simulink model "Original_example1_cs"  (R2018b)
settings: Solver=ode5  StartTime=0.0  StopTime=inf  FixedStep=1/20  RelTol=1e-3
PreLoadFcn:
  | mbxruntime.callbacks.PreLoadFcn(bdroot);
PostLoadFcn:
  | mbxruntime.callbacks.PostLoadFcn(bdroot);
InitFcn:
  | mbxruntime.callbacks.InitFcn(bdroot);
StartFcn:
  | mbxruntime.callbacks.StartFcn(bdroot);
StopFcn:
  | mbxruntime.callbacks.StopFcn(bdroot);
model workspace: external: MAT-File example1_cs_hws.mat (data not in the file)
undefined symbols (not defined in the file or in its folder): Broadcast, CameraTimestamp, Confidence, ConfidenceType, DiscIntNeverNeededParam, ErrorCode, Header, Height, Id, Id_SL_Info, InitImageOutputDir, Length, LidarTimestamp, PerceptionObstacle, PerceptionObstacle_SL_Info, PolygonPoint, PolygonPoint_SL_Info, Pose, Position, RadarTimestamp, S, SequenceNum, Theta, Timestamp, TimestampSec, TrackingTime, Type, Velocity, warningInitialVelocity, Waypoint, Waypoint_SL_Info, Width, X, x0, Y, Z
libraries: simulink x27, PreScanSimulinkLibrary x14, robotlib x12, simulink_extras x5, robotcorelib x2
(part 1 of 5)
CloseFcn:
  | mbxruntime.callbacks.CloseFcn(bdroot);
settings Model: Creator=PRESCAN  LastModifiedBy=im-lab
settings DataIOCC: LimitDataPoints=on  SaveFormat=Array  SignalLoggingSaveFormat=ModelDataLogs
settings OptimizationCC: ExpressionDepthLimit=2147483647  InitFltsAndDblsToZero=on  LifeSpan=inf
settings DebuggingCC: SaveWithParameterizedLinksMsg=none  UnderspecifiedInitializationDetection=Classic  MergeDetectMultiDrivingBlocksExec=none  SignalResolutionControl=TryResolveAllWithWarning  MultiTaskDSMMsg=warning  MultiTaskCondExecSysMsg=none  FcnCallInpInsideContextMsg=warning  StateNameClashWarn=warning  SFUnexpectedBacktrackingDiag=warning  SFNoUnconditionalDefaultTransitionDiag=warning  SFExecutionAtInitializationDiag=none
settings HardwareCC: ProdBitPerPointer=32  ProdBitPerSizeT=32  ProdBitPerPtrDiffT=32  ProdLargestAtomicFloat=None  ProdIntDivRoundTo=Undefined  ProdEndianess=Unspecified  ProdWordSize=32  ProdHWDeviceType=32-bit Generic
settings ModelReferenceCC: UpdateModelReferenceTargets=IfOutOfDate  PropagateSignalLabelsOutOfModel=off
settings SFSimCC: SimUseLocalCustomCode=off  SimParseCustomCode=off
settings SFSimCC: SimCustomHeaderCode=|
  | #include "prescan.h"
  | #include "prescan_platform.h"
settings RTWCC: RTWUseLocalCustomCode=off
settings CodeAppCC: StateflowObjectComments=on
settings GRTTargetCC: TargetFcnLib=ansi_tfl_tmw.mat  TargetLangStandard=C89/C90 (ANSI)  GeneratePreprocessorConditionals=Disable all  CombineOutputUpdateFcns=off  GRTInterface=on
settings ConfigComp: CovMetricSettings=dw  CovHtmlReporting=on  CovSaveCumulativeToWorkspaceVar=on  CovSaveSingleToWorkspaceVar=on  CovExternalEMLEnable=off

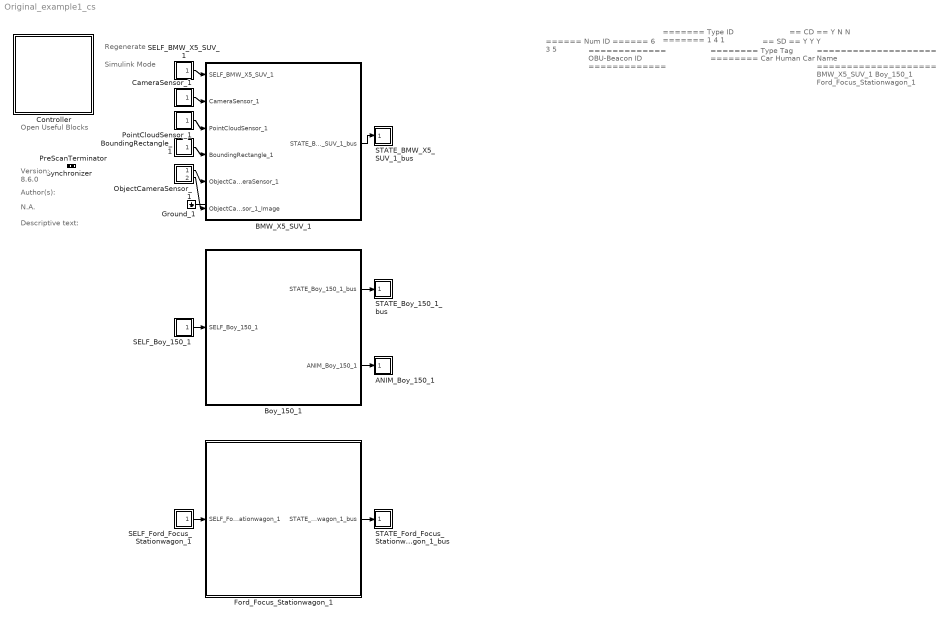
== system Original_example1_cs ==
  note: Regenerate
  note: Simulink Mode
  note: Open Useful Blocks
  note: 8.6.0
  note: Version:
  note: Author(s):
  note: N.A.
  note: Descriptive text:
  note: ======
      | Num ID
      | ======
      | 6
      | 3
      | 5
  note: =============
      | OBU-Beacon ID
      | =============
  note: =======
      | Type ID
      | =======
      | 1
      | 4
      | 1
  note: ========
      | Type Tag
      | ========
      | Car
      | Human
      | Car
  note: ==
      | SD
      | ==
      | Y
      | Y
      | Y
  note: ==
      | CD
      | ==
      | Y
      | N
      | N
  note: ====================
      | Name
      | ====================
      | BMW_X5_SUV_1
      | Boy_150_1
      | Ford_Focus_Stationwagon_1
  ANIM_Boy_150_1 : Subsystem  Tag=actuator/AnimationOutport  Priority=0  LoadFcn=load('PreScanAnimActuatorData.mat')  mask(PreScan Sink Block: State Animation){}
      mask help: The Human Animation port allows the human to walk, run or bend
      settings: OpenFcn=open_system([gcb '/Actuator'],'mask')
      mask Help: eval('openHelp(239)')
      mask Display: image(imread('HumanAnimated.jpg'))
  BMW_X5_SUV_1 : Subsystem  Tag=WorldObjectSubSystem  InitFcn=UniqueId = '35';
      mask init:
      | modelPath = GenericModelHelper.getGenericModelFilePath('ModelDepo','Vehicles\BMW_X5\BMW_X5.pgmb','cea918691563e9ae3e6a88ec95e6726a');imagePath = GenericModelHelper.getCompilationPicture(modelPath, 'BMW_X5_HighPoly.png');
      mask Display: image(imread(imagePath));color('white');text(0, 0, ' ID=6\n')
  BoundingRectangle_1 : Subsystem  Tag=sensor/BRS  Priority=3  LoadFcn=load('PrescanBRSData.mat');load('PrescanBRSMessage.mat')  mask(PreScan Source Block: Bounding Rectangle Sensor){}
      mask help: The Bounding Rectangle Sensor provides information of whereabouts of objects in images.
      settings: OpenFcn=open_system([gcb '/Sensor'],'mask')
      mask Help: eval('openHelp(1462)')
      mask Display: image(imread('BoundingRectangleSensorSL.png'))
  Boy_150_1 : Subsystem  Tag=WorldObjectSubSystem  InitFcn=UniqueId = '120';
      mask init:
      | modelPath = GenericModelHelper.getGenericModelFilePath('ModelDepo','Humans\Boy_150\Boy_150.pgmb','841f6aedbf99f0bd20b712839b1c33a7');imagePath = GenericModelHelper.getCompilationPicture(modelPath, 'Boy_150.png');
      mask Display: image(imread(imagePath));color('white');text(0, 0, ' ID=3\n')
  CameraSensor_1 : Subsystem  Tag=sensor/Camera/CameraSensor  Priority=3  mask(PreScan Source Block: Camera Sensor){}
      mask help: The Camera Sensor provides a color or monochrome image.
      settings: OpenFcn=open_system([gcb '/Sensor'],'mask')
      mask Help: eval('openHelp(457)')
      mask Display: image(imread('CameraSensor.png'))
  Controller : Subsystem  Description=193591AABAB723D448F28EC02D1309BC2290EA2C51FE96CBCBC842FCD2A763E3  Priority=-1  LoadFcn=load PreScanControllerData  mask(PreScan Simulation Controller){prescanversion='8.6.0', ModelReferencing=off, TimeStep=1/20, ControlMode=0, PreScanExecutionMode=on, ControllerCount=0, ControllerIndex=0, ControllerOptions=''}
      mask prompts: prescanversion "PreScan Version"; ModelReferencing "Use Model Referencing"; TimeStep "Upload Period [s]"; ControlMode "Control Mode"; PreScanExecutionMode "Execution Mode"; ControllerCount "Controller Count"; ControllerIndex "Controller Index"; ControllerOptions "Controller Options"
      mask help:
      | Please do not remove this block from the compilation sheet,
      | as it connects the model to the PreScan environment.
      mask init:
      | model = bdroot(gcb);
      | ExperimentFile = mbxruntime.findExperimentFile(model,true); %relative path
      | 
      | [d1, d2, d3, prescandata] = prescan_Settings();
      | ModelDepo = fullfile(prescandata,'ModelDepo'); 
      | 
      | RTmode = mbxruntime.getRTMode(model);
      | 
      | SimulationMode = get_param(bdroot,'SimulationMode');
      | if strcmp(SimulationMode, 'rapid-accelerator')
      |     SimulationMode = 'external';
      | end
      | TargetName = get_param(bdroot,'SystemTargetFile');
      settings: ModelCloseFcn=assignin('base',['model_closed_' bdroot],true);
      mask Help: eval('openHelp(812)')
      mask Display: image(imread('prescanlogo.ico'))
  Ford_Focus_Stationwagon_1 : Subsystem  Tag=WorldObjectSubSystem  InitFcn=UniqueId = '232';
      mask init:
      | modelPath = GenericModelHelper.getGenericModelFilePath('ModelDepo','Vehicles\Ford_Focus_Wagon\Ford_Focus_Wagon.pgmb','9f2f84850ce6f49365560c3439563633');imagePath = GenericModelHelper.getCompilationPicture(modelPath, 'Ford_Focus_Wagon_HighPoly.png');
      mask Display: image(imread(imagePath));color('white');text(0, 0, ' ID=5\n')
  Ground_1 : Ground
  ObjectCameraSensor_1 : Subsystem  Tag=sensor/ObjectCamera/data  Priority=3  LoadFcn=load('PrescanOCSData.mat');load('PrescanOCSMessage.mat')  mask(PreScan Source Block: Object Camera Sensor){}
      mask help: The Object Camera Sensor provides information on objects locations.
      settings: OpenFcn=open_system([gcb '/Sensor'],'mask')
      mask Help: eval('openHelp(2401)')
      mask Display: image(imread('ObjectCameraSensorSL.png'))
  PointCloudSensor_1 : Subsystem  Tag=sensor/PointCloudInport  Priority=3  mask(PreScan Source Block: Point Cloud Sensor){}
      mask help: The Point Cloud Sensor provides XYZ positions relative to the sensor
      settings: OpenFcn=open_system([gcb '/Sensor'],'mask')
      mask Help: eval('openHelp(6400)')
      mask Display: image(imread('PointCloudSensorSL.png'))
  PreScanTerminator : Subsystem  Tag=PreScanTerminator  Priority=999  LoadFcn=load PrescanTerminatorData  mask(PreScan Simulation Terminator){TimeStep=1/20}
      mask prompts: TimeStep "Upload Period [s]"
      mask help:
      | Please do not remove this block from the compilation sheet as it
      | connects the model to the PreScan environment.
      mask Help: eval('openHelp(812)')
      mask Display: image(imread('prescanlogo.ico'))
  SELF_BMW_X5_SUV_1 : Subsystem  Tag=sensor/SelfPort  Priority=3  LoadFcn=load('PreScanSelfSensorData.mat')  mask(PreScan Source Block: SELF){}
      mask help:
      | The SELF port shows (state) information of the actor itself. The outputs are position in the experiment's axis system and the GPS coordinates, and the object's absolute velocity and compass heading.
      |
      | For more information, please click Help.
      settings: OpenFcn=open_system([gcb '/Sensor'],'mask')
      mask Help: eval('openHelp(462)')
      mask Display: image(imread('GPS.png'))
  SELF_Boy_150_1 : Subsystem  Tag=sensor/SelfPort  Priority=3  LoadFcn=load('PreScanSelfSensorData.mat')  mask(PreScan Source Block: SELF){}
      mask help:
      | The SELF port shows (state) information of the actor itself. The outputs are position in the experiment's axis system and the GPS coordinates, and the object's absolute velocity and compass heading.
      |
      | For more information, please click Help.
      settings: OpenFcn=open_system([gcb '/Sensor'],'mask')
      mask Help: eval('openHelp(462)')
      mask Display: image(imread('GPS.png'))
  SELF_Ford_Focus_Stationwagon_1 : Subsystem  Tag=sensor/SelfPort  Priority=3  LoadFcn=load('PreScanSelfSensorData.mat')  mask(PreScan Source Block: SELF){}
      mask help:
      | The SELF port shows (state) information of the actor itself. The outputs are position in the experiment's axis system and the GPS coordinates, and the object's absolute velocity and compass heading.
      |
      | For more information, please click Help.
      settings: OpenFcn=open_system([gcb '/Sensor'],'mask')
      mask Help: eval('openHelp(462)')
      mask Display: image(imread('GPS.png'))
  STATE_BMW_X5_SUV_1_bus : Subsystem  Tag=actuator/StatePort  Priority=0  LoadFcn=load('PreScanStateActuatorData.mat')  mask(PreScan Sink Block: State){}
      mask help:
      | The Actor State contains a vector signal of size (9x1), containing the following signals:
      |
      | -  Position    	(x,y,z)             	[m]
      | -  Velocity    	(vx,vy,vz)         	[m/s]
      | -  Angles       	(Roll, Pitch, Yaw)	[rad]
      |
      | The Actor state is defined in the global axis system.
      | The state is superponed on the Initial position defined in the GUI.
      |
      | For more information, please click Help.
      settings: OpenFcn=open_system([gcb '/Actuator'],'mask')
      mask Help: eval('openHelp(222)')
      mask Display: image(imread('State.png'))
  STATE_Boy_150_1_bus : Subsystem  Tag=actuator/StatePort  Priority=0  LoadFcn=load('PreScanStateActuatorData.mat')  mask(PreScan Sink Block: State){}
      mask help:
      | The Actor State contains a vector signal of size (9x1), containing the following signals:
      |
      | -  Position    	(x,y,z)             	[m]
      | -  Velocity    	(vx,vy,vz)         	[m/s]
      | -  Angles       	(Roll, Pitch, Yaw)	[rad]
      |
      | The Actor state is defined in the global axis system.
      | The state is superponed on the Initial position defined in the GUI.
      |
      | For more information, please click Help.
      settings: OpenFcn=open_system([gcb '/Actuator'],'mask')
      mask Help: eval('openHelp(222)')
      mask Display: image(imread('State.png'))
  STATE_Ford_Focus_Stationwagon_1_bus : Subsystem  Tag=actuator/StatePort  Priority=0  LoadFcn=load('PreScanStateActuatorData.mat')  mask(PreScan Sink Block: State){}
      mask help:
      | The Actor State contains a vector signal of size (9x1), containing the following signals:
      |
      | -  Position    	(x,y,z)             	[m]
      | -  Velocity    	(vx,vy,vz)         	[m/s]
      | -  Angles       	(Roll, Pitch, Yaw)	[rad]
      |
      | The Actor state is defined in the global axis system.
      | The state is superponed on the Initial position defined in the GUI.
      |
      | For more information, please click Help.
      settings: OpenFcn=open_system([gcb '/Actuator'],'mask')
      mask Help: eval('openHelp(222)')
      mask Display: image(imread('State.png'))
  Synchronizer : Subsystem  Tag=PreScanSynchronizer  Priority=1  LoadFcn=load PrescanSynchronizeData  mask(PreScan Simulation Core Block){TimeStep=1/20}
      mask prompts: TimeStep "Timestep [s]"
      mask help:
      | Please do not remove this block from the PreScan compilation sheet,
      | as it contains essential configuration parameters for a PreScan simulation.
      settings: DeleteFcn=PreScanBlockDeleteFcn;
      mask Display: image(imread('prescanlogo.ico'))
  wires:
  BMW_X5_SUV_1/1(STATE_BMW_X5_SUV_1_bus) -> STATE_BMW_X5_SUV_1_bus/1(STATE_BMW_X5_SUV_1_bus)
  SELF_BMW_X5_SUV_1/1(SELF_BMW_X5_SUV_1) -> BMW_X5_SUV_1/1(SELF_BMW_X5_SUV_1)
  CameraSensor_1/1(CameraSensor_1) -> BMW_X5_SUV_1/2(CameraSensor_1)
  BoundingRectangle_1/1(BoundingRectangle_1) -> BMW_X5_SUV_1/4(BoundingRectangle_1)
  ObjectCameraSensor_1/1(ObjectCameraSensor_1) -> BMW_X5_SUV_1/5(ObjectCameraSensor_1)
  ObjectCameraSensor_1/2(ObjectCameraSensor_1_Image) -> BMW_X5_SUV_1/6(ObjectCameraSensor_1_Image)
  Boy_150_1/1(STATE_Boy_150_1_bus) -> STATE_Boy_150_1_bus/1(STATE_Boy_150_1_bus)
  Boy_150_1/2(ANIM_Boy_150_1) -> ANIM_Boy_150_1/1(ANIM_Boy_150_1)
  SELF_Boy_150_1/1(SELF_Boy_150_1) -> Boy_150_1/1(SELF_Boy_150_1)
  Ford_Focus_Stationwagon_1/1(STATE_Ford_Focus_Stationwagon_1_bus) -> STATE_Ford_Focus_Stationwagon_1_bus/1(STATE_Ford_Focus_Stationwagon_1_bus)
  SELF_Ford_Focus_Stationwagon_1/1(SELF_Ford_Focus_Stationwagon_1) -> Ford_Focus_Stationwagon_1/1(SELF_Ford_Focus_Stationwagon_1)
  PointCloudSensor_1/1(PointCloudSensor_1) -> BMW_X5_SUV_1/3(PointCloudSensor_1)
  Ground_1/1 -> ?

== system Original_example1_cs/ANIM_Boy_150_1 ==
  ANIM_Boy_150_1 : Inport  Tag=inport/AnimationOutport  OutDataTypeStr=Bus: PRESCAN_ANIMACTUATORDATA  PortDimensions=1  SampleTime=1/20  BusOutputAsStruct=on
  Actuator : S-Function  FunctionName=sfun_AnimActuator  Parameters=UniqueID, TimeStep  SFunctionDeploymentMode=off  EnableBusSupport=off  mask(PreScan Sink Block: State Animation){UniqueID=120, TimeStep=1/20}
      mask prompts: UniqueID "Auto-Assigned: Unique ID"; TimeStep "Auto-Assigned: Upload Period [s]"
      mask help: The Human Animation port allows the human to walk, run or bend
      mask Help: eval('openHelp(239)')
      mask Display: image(imread('HumanAnimated.jpg'))
  wires:
  ANIM_Boy_150_1/1 -> Actuator/1

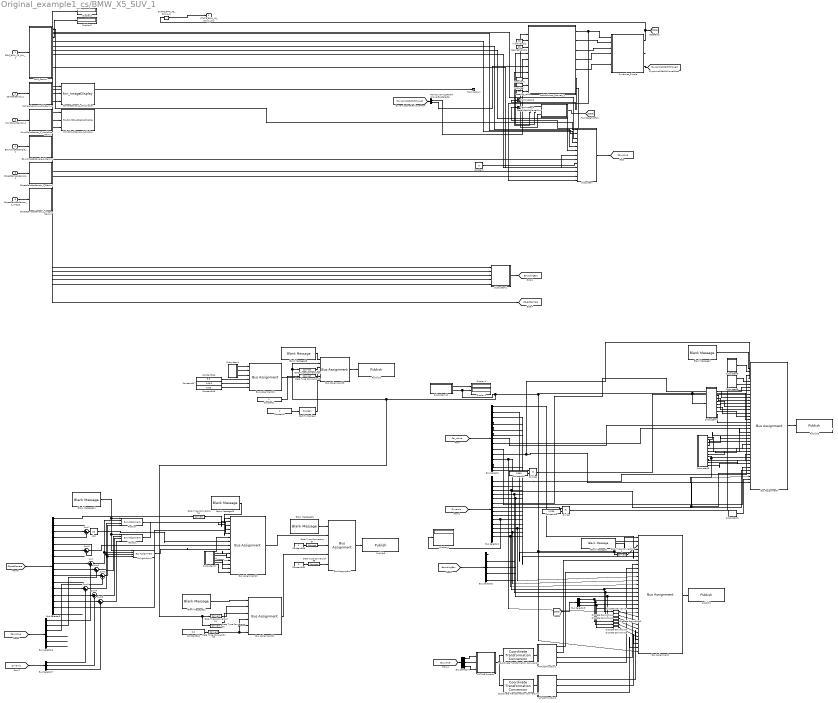
== system Original_example1_cs/BMW_X5_SUV_1 ==
  note: 0
  SELF_BMW_X5_SUV_1 : Inport  Tag=inport/SelfPort  OutDataTypeStr=Bus: PRESCAN_SELFSENSORDATA  PortDimensions=1  SampleTime=1/20  BusOutputAsStruct=on
  CameraSensor_1 : Inport  Tag=inport/Camera/CameraSensor  Port=2  OutDataTypeStr=uint8  SampleTime=1/20  BusOutputAsStruct=on
  PointCloudSensor_1 : Inport  Tag=inport/PointCloudInport  Port=3  OutDataTypeStr=single  SampleTime=1/20  BusOutputAsStruct=on
  BoundingRectangle_1 : Inport  Tag=inport/BRS  Port=4  OutDataTypeStr=Bus: PRESCAN_BRS_MESSAGE  PortDimensions=32  SampleTime=1/20  BusOutputAsStruct=on
  ObjectCameraSensor_1 : Inport  Tag=inport/ObjectCamera/data  Port=5  OutDataTypeStr=Bus: PRESCAN_OCS_MESSAGE  PortDimensions=1  SampleTime=1/20  BusOutputAsStruct=on
  ObjectCameraSensor_1_Image : Inport  Tag=inport/ObjectCamera/image  Port=6  OutDataTypeStr=uint8  SampleTime=1/20  BusOutputAsStruct=on
  Abs : Abs
  Blank Message1 : robotlib/Blank Message  messageClass=Message  entityType=my_msgs/LocalizationEstimate  messageType=my_msgs/LocalizationEstimate  SampleTime=inf
      settings: SourceProductBaseCode=RO
  Blank Message19 : robotlib/Blank Message  messageClass=Message  entityType=my_msgs/RoutingRequest  messageType=my_msgs/RoutingRequest  SampleTime=inf
      settings: SourceProductBaseCode=RO
  Blank Message22 : robotlib/Blank Message  messageClass=Message  entityType=my_msgs/Header  messageType=my_msgs/Header  SampleTime=inf
      settings: SourceProductBaseCode=RO
  Blank Message23 : robotlib/Blank Message  messageClass=Message  entityType=my_msgs/PerceptionObstacle  messageType=my_msgs/PerceptionObstacle  SampleTime=inf
      settings: SourceProductBaseCode=RO
  Blank Message24 : robotlib/Blank Message  messageClass=Message  entityType=my_msgs/Point3D  messageType=my_msgs/Point3D  SampleTime=inf
      settings: SourceProductBaseCode=RO
  Blank Message25 : robotlib/Blank Message  messageClass=Message  entityType=my_msgs/PerceptionObstacles  messageType=my_msgs/PerceptionObstacles  SampleTime=inf
      settings: SourceProductBaseCode=RO
  Blank Message7 : robotlib/Blank Message  messageClass=Message  entityType=my_msgs/Chassis  messageType=my_msgs/Chassis  SampleTime=inf
      settings: SourceProductBaseCode=RO
  BoundingRectangle_1_Demux : Subsystem  Tag=demux/BRS  mask(PreScan Demux Block: Bounding Rectangle Sensor){detectableObjects=32}
      mask prompts: detectableObjects "Max. detectable objects"
      settings: DeleteFcn=PreScanBlockDeleteFcn;
      mask Help: eval('openHelp(1462)')
      mask Display:
      | port_label('input', 1, 'BRS')
      | port_label('output', 1, 'Object ID')
      | port_label('output', 2, 'Left')
      | port_label('output', 3, 'Right')
      | port_label('output', 4, 'Bottom')
      | port_label('output', 5, 'Top')
  Bus Assignment : BusAssignment  AssignedSignals=PerceptionObstacle,PerceptionObstacle_SL_Info.CurrentLength,Header,ErrorCode
  Bus Assignment1 : BusAssignment  AssignedSignals=Header.TimestampSec,Header.SequenceNum,Pose.Position.X,Pose.Position.Y,Pose.Position.Z,Pose.Orientation.Qx,Pose.Orientation.Qy,Pose.Orientation.Qz,Pose.Orientation.Qw,Pose.LinearVelocity.X,Pose.LinearVelocity.Y,Pose.LinearVelocity.Z,Pose.LinearAccelration.X,Pose.LinearAccelration.Y,Pose.LinearAccelration.Z,Pose.AngularVelocity.X,Pose.AngularVelocity.Y,Pose.AngularVelocity.Z,Pose.Heading,Pose.LinearAccelerationVrf.X,Pose.LinearAccelerationVrf.Y,Pose.LinearAccelerationVrf.Z,Pose.AngularAccelerationVrf.X,Pose.AngularAccelerationVrf.Y,Pose.AngularAccelerationVrf.Z,Pose.EulerAngles.X,Pose.EulerAngles.Y,Pose.EulerAngles.Z,MeasurementTime
  Bus Assignment19 : BusAssignment  AssignedSignals=Header.TimestampSec,Header.SequenceNum,Waypoint,Waypoint_SL_Info.CurrentLength,Broadcast
  Bus Assignment21 : BusAssignment  AssignedSignals=Id,Id_SL_Info.CurrentLength,S,Pose.X,Pose.Y
  Bus Assignment22 : BusAssignment  AssignedSignals=TimestampSec,SequenceNum,LidarTimestamp,CameraTimestamp,RadarTimestamp
  Bus Assignment23 : BusAssignment  AssignedSignals=Id,Position,Theta,Velocity,Length,Width,Height,PolygonPoint,TrackingTime,Type,Timestamp,Confidence,ConfidenceType,PolygonPoint_SL_Info.CurrentLength
  Bus Assignment7 : BusAssignment  AssignedSignals=EngineStarted,EngineRpm,SpeedMps,OdometerM,FuelRangeM,ThrottlePercentage,BrakePercentage,SteeringPercentage,ParkingBrake,HighBeamSignal,LowBeamSignal,LeftTurnSignal,RightTurnSignal,Wiper,DrivingMode,Header.TimestampSec,Header.SequenceNum,ChassisGps.Latitude,ChassisGps.Longitude,ChassisGps.GpsValid,ChassisGps.Year,ChassisGps.Month,ChassisGps.Day,ChassisGps.Hours,ChassisGps.Minutes,ChassisGps.Seconds,ChassisGps.CompassDirection,ChassisGps.Pdop,ChassisGps.IsGpsFault,ChassisGps.IsInferred,ChassisGps.Altitude,ChassisGps.Heading,ChassisGps.Hdop,ChassisGps.Vdop,ChassisGps.NumSatellites,ChassisGps.GpsSpeed
  Bus Selector : BusSelector  OutputSignals=x,y,z,Rotx,Roty,Rotz,GPS Latitude,GPS Longitude,GPS Altitude,Velocity,Heading Angle,Yaw rate,steer[deg]
  Bus Selector1 : BusSelector  OutputSignals=NEngine_[rpm],Gear_[-],Ax_[ms-2],Ay_[ms-2],Az_[ms-2],Throttle_[perc],Brake_[bar],PEngine_[kW],PDrive_[kW],Roll_[deg],Pitch_[deg],vx_[ms-1],vy_[ms-1],vz_[ms-1]
  Bus Selector2 : BusSelector  OutputSignals=Object ID,Left,Right,Bottom,Top
  Bus Selector3 : BusSelector  OutputSignals=AngularVelocityRoll,AngularVelocityPitch,AngularVelocityYaw
  Bus Selector4 : BusSelector  OutputSignals=Rotx,Roty,Rotz
  Bus Selector5 : BusSelector  OutputSignals=Object ID[-],ObjectTypeID[-],Left[-],Right[-],Bottom[-],Top[-],Range[m],RangeX[m],RangeY[m],RangeZ[m],DopplerVelocity[ms-1],DopplerVelocityX[ms-1],DopplerVelocityY[ms-1],DopplerVelocityZ[ms-1],Theta[deg],Phi[deg]
  Bus Selector6 : BusSelector  OutputSignals=x,y,z,Rotx,Roty,Rotz
  Bus Selector7 : BusSelector  OutputSignals=vx_[ms-1],vy_[ms-1],vz_[ms-1]
  CameraSensor_1_CM_Demux : Subsystem  Tag=demux/Camera/Color  mask{SensorName=CameraSensor_1, hres=320, vres=240}
      mask prompts: SensorName "Sensor Name"; hres "Horizontal Resolution"; vres "Vertical Resolution"
      mask Help: eval('openHelp(457)')
      mask Display:
      | fprintf('MONO CAMERA:\n Color\n %s \n %d x %d px',SensorName,hres,vres)
      | port_label('output',1,'R')
      | port_label('output',2,'G')
      | port_label('output',3,'B')
  CameraSensor_1_CM_Display : M-S-Function  Tag=CameraSensor_Color_Display  InitFcn=InitImageOutputDir(gcb);  FunctionName=fcn_ImageDisplay  Parameters=SensorName EnableDisplay EnablePosition DisplayPosition FigureHandle SaveResults BitmapFormat TempOutputDir CameraType DataType  mask(PreScan Color Display Block){SensorName=CameraSensor_1, EnableDisplay=on, EnablePosition=off, DisplayPosition=[10 10 320 240], FigureHandle=3501, SaveResults=off, Format=PNG, TempOutputDir=0, CameraType=Mono, DataType=uint8}
      mask prompts: SensorName "User Specified: Title of Display"; EnableDisplay "Active"; EnablePosition "Set Display window position"; DisplayPosition "Display window position [xpos ypos width height]"; FigureHandle "Unique Handle"; SaveResults "Save results"; TempOutputDir "OutputDir"; CameraType "Camera Type"; DataType "Image Data Type"
      mask help: This block displays the RGB output of a PreScan camera sensor.
      mask init:
      | if EnableDisplay
      |     EnableString='';
      |     EnableColor='gray';
      | else
      |     EnableString='INACTIVE';
      |     EnableColor='red';
      | end
      | switch Format
      |     case 1
      |         BitmapFormat = 'png';
      |     case 2
      |         BitmapFormat = 'bmp';
      |     case 3
      |         BitmapFormat = 'jpg';
      | end 
      | if CameraType==1
      |     CameraTypeName='MONO';
      |     PortNumber=0;
      | else
      |     CameraTypeName='STEREO';
      |     PortNumber=3;
      | end
      settings: CopyFcn=CopyFcnDisplay  DeleteFcn=PreScanBlockDeleteFcn;  ModelCloseFcn=fcn_ImageDisplay_ModelCloseFcn
      mask Help: eval('openHelp(457)')
      mask Callback EnablePosition:
      | MV=get_param(gcb,'MaskVisibilities');
      | if strcmp(get_param(gcb,'EnablePosition'),'on')
      |     MV{4}='on';
      | else
      |     MV{4}='off';
      | end
      | set_param(gcb,'MaskVisibilities',MV);
      | clear MV;
      mask TypeOptions Format: PNG | BMP | JPG
      mask TypeOptions CameraType: Mono | Stereo
      mask TypeOptions DataType: uint8 | single
      mask Display:
      | color(EnableColor);
      | fprintf('%s\n DISPLAY:\n Color \n %s',EnableString,SensorName)
      | port_label('input',1,'R')
      | port_label('input',2,'G')
      | port_label('input',3,'B')
      | port_label('input',PortNumber+1,'R')
      | port_label('input',PortNumber+2,'G')
      | port_label('input',PortNumber+3,'B')
  Cast To Boolean : DataTypeConversion  OutDataTypeStr=boolean
  Constant : Constant  Value=0
  Constant1 : Constant
  Constant15 : Constant  Value=1/150
  Constant16 : Constant  Value=1/360
  Constant2 : Constant
  Constant346 : Constant  Value=5.3
  Constant347 : Constant  Value=146.5
  Constant348 : Constant  Value=0.69
  Constant352 : Constant  Value=0
  Constant358 : Constant
  Constant361 : Constant  Value=0.0
  Coordinate Transformation Conversion : robotcorelib/Coordinate Transformation Conversion  InputRepresentation=Rotation Matrix  InputEulerSequence=ZYX  ShowTrVecInputPort=on  OutputRepresentation=Quaternion  OutputEulerSequence=ZYX  ShowTrVecOutputPort=on  SimulateUsing=Interpreted execution
      settings: SourceProductBaseCode=RO
  Coordinate Transformation Conversion1 : robotcorelib/Coordinate Transformation Conversion  InputRepresentation=Rotation Matrix  InputEulerSequence=ZYX  ShowTrVecInputPort=on  OutputRepresentation=Euler Angles  OutputEulerSequence=XYZ  ShowTrVecOutputPort=on  SimulateUsing=Interpreted execution
      settings: SourceProductBaseCode=RO
  Data Type Conversion{1..2,90..95,97} (9 alike) : DataTypeConversion
  DesiredVelocity : Constant  Tag=DesiredVelocity  Value=15
  Discrete Derivative{,1..5} (6 alike) : simulink/Discrete/Discrete Derivative  gainval=1.0  ICPrevScaledInput=0.0  OutMin=[]  OutMax=[]  OutDataType=fixdt(1, 16)  OutScaling=2^-10  DoSatur=off
  Display{1..5} (5 alike) : Display
  Divide : Product  Inputs=**
  Divide1 : Product  Inputs=**
  Dynamics_Simple : Subsystem  Tag=Simple_Vehicle_Dynamics  mask(PreScan Block: Simple Dynamics){Migrate=on, TimeStep=1/20, ComputationMode=Continuous_Time, initialX=69.6504, initialY=66.9207, initialZ=0.69, initialRoll=0, initialPitch=0, initialYaw=0.044635}
      mask prompts: Migrate "Migrate. During migration this block will be replaced by a newer one."; TimeStep "Auto assigned: Time Step [s]"; ComputationMode "Computation mode:"; initialX "Ini x-position VEHICLE wrt GLOBAL axis system [m]"; initialY "Ini y-position VEHICLE wrt GLOBAL axis system [m]"; initialZ "Ini z-position VEHICLE wrt GLOBAL axis system [m]"; initialRoll "Ini roll-angle BODY wrt VEHICLE axis system [deg]"; initialPitch "Ini pitch-angle BODY wrt VEHICLE axis system [deg]"; initialYaw "Ini yaw-angle VEHICLE wrt GLOBAL axis system [deg]"
      mask help:
      | The Simple Dynamics Model is selected in the GUI to simulate vehicle dynamics behavior.
      |
      | The Simple Dynamics Model is completely open to the user. The parameters of this model can be set in the Simple Dynamics dialog in the GUI.
      |
      | For more information, please click Help.
      mask init:
      | p = SimpleDyn_pars;
      settings: DeleteFcn=PreScanBlockDeleteFcn;
      mask Help: eval('openHelp(220)')
      mask Display:
      | image(imread('SimpleDyn.png'))
      | port_label('input', 1, '{\delta}_S_t_ _e_e_r [deg]','texmode','on')
      | port_label('input', 2, 'Throttle [%]')
      | port_label('input', 3, 'Brake Pres [bar]')
      | port_label('input', 4, 'V_0 [ms-1]','texmode','on')
      | port_label('input', 5, 'Auto=[0]/Manual=[1]')
      | port_label('input', 6, 'Auto_GearShift')
      | port_label('input', 7, 'Manual_GearShift')
      | port_label('output', 1, 'State')
      | port_label('output', 2, 'Vx [ms-1]')
      | port_label('output', 3, 'Perf Params')
  FromDynamics2PathFollowerBusSelector : BusSelector  OutputSignals=vx_[ms-1],vy_[ms-1]
  InitialVelocity : Constant  Tag=InitialVelocity  Value=15
  MATLAB Function : MATLAB Function  TreatAsAtomicUnit=on
  MATLAB Function1 : MATLAB Function  TreatAsAtomicUnit=on
  MATLAB Function2 : MATLAB Function  TreatAsAtomicUnit=on
  ObjectCameraSensor_1_Demux : Subsystem  Tag=demux/OCS  mask(PreScan Demux Block: Object Camera Sensor){detectableObjects=1}
      mask prompts: detectableObjects "Max. detectable objects"
      settings: DeleteFcn=PreScanBlockDeleteFcn;
      mask Help: eval('openHelp(2401)')
      mask Display:
      | port_label('input', 1, 'OCS')
      | port_label('output', 1, 'OCS Data')
  ObjectCameraSensor_1_Image_Demux : Subsystem  Tag=demux/Camera/Color  mask{SensorName=ObjectCameraSensor_1, hres=320, vres=240}
      mask prompts: SensorName "Sensor Name"; hres "Horizontal Resolution"; vres "Vertical Resolution"
      mask Help: eval('openHelp(2401)')
      mask Display:
      | fprintf('MONO CAMERA:\n Color\n %s \n %d x %d px',SensorName,hres,vres)
      | port_label('output',1,'R')
      | port_label('output',2,'G')
      | port_label('output',3,'B')
  PathFollower_Preview_1 : Subsystem  Tag=PathFollower_Preview  mask(PreScan Block: Path Follower with Preview){Migrate=on, LongCtrl_P=20, LongCtrl_I=0.3, LongCtrl_D=3.065, LongCtrl_AWU=1, LongCtrlDefault_P=20, LongCtrlDefault_I=0.3, LongCtrlDefault_D=3.065, LongCtrlDefault_AWU=1, PathUniqueID=109, mass=2220, Jzz=4193, length_a=2.82 - 1.69, length_l=2.82, Angle_Max_SteeringWheel=500, PreviewTime=1, DelayTime=0.1, LowSpeedLimit=20, MaxSteeringRate=1200, CSSampleTime=1/20, PFIntegrationFrequency=20}
      mask prompts: Migrate "Migrate. During migration this block will be replaced by a newer one."; LongCtrl_P "Longitudinal Controller P"; LongCtrl_I "Longitudinal Controller I"; LongCtrl_D "Longitudinal Controller D"; LongCtrl_AWU "Longitudinal Controller AWU"; PathUniqueID "Path Unique ID"; mass "Mass vehicle total [kg]"; Jzz "Inertia vehicle around yaw axis [kg m2]"; length_a "Distance between COG and front axle [m]"; length_l "Length of wheelbase [m]"; Angle_Max_SteeringWheel "Maximum steering wheel angle [deg]"; PreviewTime "Preview time [s]"; DelayTime "Delay time [s]"; LowSpeedLimit "Low-speed limit [km/h]"; MaxSteeringRate "Maximum steering wheel angle rate [deg/s]"; CSSampleTime "Compilation Sheet sample time [s]"; PFIntegrationFrequency "Lateral controller frequency [Hz]"
      mask help:
      | The Path Follower Model is selected in the GUI to simulate driver behavior.
      |
      | For more information, please click Help.
      mask init:
      | RefreshCounter = max(floor((1/CSSampleTime) / (PFIntegrationFrequency)), 1);
      | PathFollowerBlockPath = gcb;
      mask Help: eval('openHelp(233)')
      mask DialogControl Container12 Prompt: Controller Parameters
      mask DialogControl Control2 Prompt: Reset PID parameters
      mask DialogControl Control2 Callback:
      | LongCtrlDefault_P = get_param(gcb,'LongCtrlDefault_P');
      | set_param(gcb,'LongCtrl_P',LongCtrlDefault_P);
      | 
      | LongCtrlDefault_I = get_param(gcb,'LongCtrlDefault_I');
      | set_param(gcb,'LongCtrl_I',LongCtrlDefault_I);
      | 
      | LongCtrlDefault_D = get_param(gcb,'LongCtrlDefault_D');
      | set_param(gcb,'LongCtrl_D',LongCtrlDefault_D);
      | 
      | LongCtrlDefault_AWU = get_param(gcb,'LongCtrlDefault_AWU');
      | set_param(gcb,'LongCtrl_AWU',LongCtrlDefault_AWU);
      mask DialogControl Container10 Prompt: System Parameters
  PointCloudSensor_1_Display : M-S-Function  Tag=PointCloudSensor_Display  FunctionName=fcn_PointCloudSensorDisplay  Parameters=SensorName EnableDisplay FigureHandle EnableIntensity  mask(PreScan Point Cloud Display Block){SensorName=PointCloudSensor_1, EnableDisplay=off, FigureHandle=3502, EnableIntensity=off}
      mask prompts: SensorName "User Specified: Title of Display"; EnableDisplay "Active"; FigureHandle "Unique Handle"; EnableIntensity "Visualize Intensity"
      mask help: This block displays world position (and intensity) output of a PreScan point cloud sensor.
      mask init:
      | if EnableDisplay
      |     EnableString='';
      |     EnableColor='gray';
      | else
      |     EnableString='INACTIVE';
      |     EnableColor='red';
      | end
      settings: DeleteFcn=PreScanBlockDeleteFcn;  ModelCloseFcn=fcn_ImageDisplay_ModelCloseFcn
      mask Help: eval('openHelp(6400)')
      mask Display:
      | color(EnableColor);
      | fprintf('%s\n PointCloud Display:\n %s',EnableString,SensorName)
      | port_label('input',1,'X')
      | port_label('input',2,'Y')
      | port_label('input',3,'Z')
      | 
      | if EnableIntensity
      |     port_label('input',4,'I')
      | end
  PointCloudSensor_1_WorldPos_Demux : Subsystem  Tag=demux/PCS/WorldPos  mask{SensorName=PointCloudSensor_1, offset=0, hres=320, vres=160}
      mask prompts: SensorName "Sensor Name"; offset "Data Start"; hres "Horizontal Resolution"; vres "Vertical Resolution"
      mask Help: eval('openHelp(6400)')
      mask Display:
      | fprintf('Point Cloud:\n Data\n %s \n %d x %d px',SensorName,hres,vres)
      | port_label('output',1,'X')
      | port_label('output',2,'Y')
      | port_label('output',3,'Z')
  PolygonPoint : BusAssignment  AssignedSignals=X,Y,Z
  "Position " : BusAssignment  AssignedSignals=X,Y,Z
  Publish1 : robotlib/Publish  topicSource=Specify your own  topic=/my_msgs/LocalizationEstimate  messageType=my_msgs/LocalizationEstimate  messageQueueLength=1
      settings: SourceProductBaseCode=RO
  Publish2 : robotlib/Publish  topicSource=Specify your own  topic=/my_msgs/RoutingRequest  messageType=my_msgs/RoutingRequest  messageQueueLength=1
      settings: SourceProductBaseCode=RO
  Publish3 : robotlib/Publish  topicSource=Specify your own  topic=/my_msgs/PerceptionObstacles  messageType=my_msgs/PerceptionObstacles  messageQueueLength=1
      settings: SourceProductBaseCode=RO
  Publish5 : robotlib/Publish  topicSource=Specify your own  topic=/my_msgs/Chassis  messageType=my_msgs/Chassis  messageQueueLength=1
      settings: SourceProductBaseCode=RO
  SELF_Demux : Subsystem  Tag=demux/SelfPort  mask(PreScan Demux Block:){}
      mask help:
      | The SELF port shows (state) information of the actor itself. The outputs are position in the experiment's axis system and the GPS coordinates, and the object's absolute velocity and compass heading.
      |
      | For more information, please click Help.
      settings: DeleteFcn=PreScanBlockDeleteFcn;
      mask Help: eval('openHelp(462)')
      mask Display:
      | port_label('output',1,'x [m]')
      | port_label('output',2,'y [m]')
      | port_label('output',3,'z [m]','texmode','on')
      | port_label('output',4,'Rotx [deg]','texmode','on')
      | port_label('output',5,'Roty [deg]','texmode','on')
      | port_label('output',6,'Rotz [deg]','texmode','on')
      | port_label('output',7,'GPS lat [deg]','texmode','on')
      | port_label('output',8,'GPS long [deg]','texmode','on')
      | port_label('output',9,'GPS alt [m]','texmode','on')
      | port_label('output',10,'Velocity [m/s]')
      | port_label('output',11,'Heading [deg]')
      | port_label('output',12,'Yaw rate [deg/s]')
  STATE_BMW_X5_SUV_1_rc : RateTransition  Tag=mux_rc/StatePort  OutPortSampleTimeOpt=Inherit
  State2PathFollowerCnv : Subsystem  Tag=State2PFConnection/cnv
  Subsystem : Subsystem
  Subsystem1 : Subsystem
  Subsystem10 : Subsystem
  Subsystem3 : Subsystem
  Subsystem4 : Subsystem
  Subsystem5 : Subsystem
  Subsystem6 : Subsystem
  Subsystem7 : Subsystem
  Subsystem8 : Subsystem
  Subsystem9 : Subsystem
  Sum{,1..5} (6 alike) : Sum  Inputs=|++
  Sum6 : Sum  Inputs=|+-
  Sum7 : Sum  Inputs=|+-
  Terminator_5 : Terminator
  Terminator_6 : Terminator
  Terminator_7 : Terminator
  Velocity : BusAssignment  AssignedSignals=X,Y,Z
  steering_ratio : Constant  Tag=steering_ratio  Value=20
  susp_front : Constant  Tag=susp_front  Value=90943
  susp_rear : Constant  Tag=susp_rear  Value=148091
  STATE_BMW_X5_SUV_1_bus : Outport  Tag=outport/StatePort  OutDataTypeStr=Bus: PRESCAN_STATEACTUATORDATA  PortDimensions=1  SampleTime=1/20
  tag scope: BoundingBox=global, Car_value=global, ObjectCamera=global
  wires:
  SELF_Demux/10(velocity [m/s]) -> Subsystem/10(In10)  "Velocity"
  SELF_Demux/11(heading [deg]) -> Subsystem/11(In11)  "Heading Angle"
  SELF_Demux/12(yaw rate [deg/s]) -> Subsystem/12(In12)  "Yaw rate"
  SELF_Demux/1(x [m]) -> Display3/1, Subsystem/1(In1)  "x"
  SELF_Demux/2(y [m]) -> Subsystem/2(In2)  "y"
  SELF_Demux/3(z [m]) -> Display5/1, Subsystem/3(In3)  "z"
  SELF_Demux/4(rotx [deg]) -> Subsystem/4(In4)  "Rotx"
  SELF_Demux/5(roty [deg]) -> Subsystem/5(In5)  "Roty"
  SELF_Demux/6(rotz [deg]) -> Subsystem/6(In6)  "Rotz"
  SELF_Demux/7(GPS lat [deg]) -> Subsystem/7(In7)  "GPS Latitude"
  SELF_Demux/8(GPS long [deg]) -> Subsystem/8(In8)  "GPS Longitude"
  Subsystem/1(Out1) -> [Car_value]
  [Car_value] -> Bus Selector/1
  Constant/1 -> Subsystem/9(In9)  "GPS Altitude"
  Bus Selector/1 -> Bus Assignment1/4  "<x>"
  Bus Selector/2 -> Bus Assignment1/5  "<y>"
  Bus Selector/3 -> Bus Assignment1/6  "<z>"
  Bus Selector/4 -> ?  "<Rotx>"
  Bus Selector/5 -> ?  "<Roty>"
  Bus Selector/6 -> ?  "<Rotz>"
  Bus Selector/7 -> Bus Assignment7/19  "<GPS Latitude>"
  Bus Selector/8 -> Bus Assignment7/20  "<GPS Longitude>"
  Bus Selector/9 -> Bus Assignment7/32  "<GPS Altitude>"
  Bus Selector/10 -> Bus Assignment7/37, Bus Assignment7/4  "<Velocity>"
  Bus Selector/11 -> Bus Assignment1/20, Bus Assignment7/33  "<Heading Angle>"
  Bus Selector/12 -> ?  "<Yaw rate>"
  [Dynamic] -> Bus Selector1/1
  Bus Selector1/1 -> Bus Assignment7/3  "<NEngine_[rpm]>"
  Bus Selector1/2 -> ?  "<Gear_[-]>"
  Bus Selector1/3 -> Discrete Derivative/1, Bus Assignment1/14  "<Ax_[ms-2]>"
  Bus Selector1/4 -> Discrete Derivative1/1, Bus Assignment1/15  "<Ay_[ms-2]>"
  Bus Selector1/5 -> Discrete Derivative2/1, Bus Assignment1/16  "<Az_[ms-2]>"
  Bus Selector1/6 -> Bus Assignment7/7  "<Throttle_[perc]>"
  Bus Selector1/7 -> Divide/1  "<Brake_[bar]>"
  Bus Selector1/8 -> ?  "<PEngine_[kW]>"
  Bus Selector1/9 -> ?  "<PDrive_[kW]>"
  Bus Selector1/10 -> Display4/1  "<Roll_[deg]>"
  Bus Selector1/11 -> ?  "<Pitch_[deg]>"
  Bus Selector1/12 -> Bus Assignment1/11  "<vx_[ms-1]>"
  Bus Selector1/13 -> Bus Assignment1/12  "<vy_[ms-1]>"
  Bus Selector1/14 -> Bus Assignment1/13  "<vz_[ms-1]>"
  BoundingRectangle_1_Demux/1(ObjectID) -> Subsystem1/1(In1)  "Object ID"
  BoundingRectangle_1_Demux/2(Left) -> Subsystem1/2(In2)  "Left"
  BoundingRectangle_1_Demux/3(Right) -> Subsystem1/3(In3)  "Right"
  BoundingRectangle_1_Demux/4(Bottom) -> Subsystem1/4(In4)  "Bottom"
  BoundingRectangle_1_Demux/5(Top) -> Subsystem1/5(In5)  "Top"
  Subsystem1/1(Out1) -> [BoundingBox]
  [BoundingBox] -> Bus Selector2/1
  Bus Selector2/2 -> ?  "<Left>"
  Bus Selector2/3 -> ?  "<Right>"
  Bus Selector2/4 -> ?  "<Bottom>"
  Bus Selector2/5 -> ?  "<Top>"
  ObjectCameraSensor_1_Demux/1(OCS Data) -> [ObjectCamera]
  [ObjectCamera] -> Bus Selector5/1
  Bus Selector5/1 -> Data Type Conversion94/1  "<Object ID[-]>"
  Bus Selector5/2 -> ?  "<ObjectTypeID[-]>"
  Bus Selector5/3 -> Sum7/1  "<Left[-]>"
  Bus Selector5/4 -> Sum7/2  "<Right[-]>"
  Bus Selector5/5 -> Sum6/2  "<Bottom[-]>"
  Bus Selector5/6 -> Sum6/1  "<Top[-]>"
  Bus Selector5/7 -> ?  "<Range[m]>"
  Bus Selector5/8 -> Sum/1  "<RangeX[m]>"
  Bus Selector5/9 -> Sum1/1  "<RangeY[m]>"
  Bus Selector5/10 -> Sum2/1  "<RangeZ[m]>"
  Bus Selector5/11 -> ?  "<DopplerVelocity[ms-1]>"
  Bus Selector5/12 -> Sum3/1  "<DopplerVelocityX[ms-1]>"
  Bus Selector5/13 -> Sum4/1  "<DopplerVelocityY[ms-1]>"
  Bus Selector5/15 -> Bus Assignment23/4  "<Theta[deg]>"
  Bus Selector5/16 -> ?  "<Phi[deg]>"
  STATE_BMW_X5_SUV_1_rc/1 -> STATE_BMW_X5_SUV_1_bus/1
  SELF_BMW_X5_SUV_1/1 -> SELF_Demux/1(SELF)
  CameraSensor_1/1 -> CameraSensor_1_CM_Demux/1(In1)
  CameraSensor_1_CM_Demux/1(R) -> CameraSensor_1_CM_Display/1
  CameraSensor_1_CM_Demux/2(G) -> CameraSensor_1_CM_Display/2
  CameraSensor_1_CM_Demux/3(B) -> CameraSensor_1_CM_Display/3
  BoundingRectangle_1/1 -> BoundingRectangle_1_Demux/1(BRS)
  ObjectCameraSensor_1/1 -> ObjectCameraSensor_1_Demux/1(OCS)
  ObjectCameraSensor_1_Image/1 -> ObjectCameraSensor_1_Image_Demux/1(In1)
  susp_front/1 -> PathFollower_Preview_1/9(CorneringStiffness_Tyres_Front [N/rad])
  susp_rear/1 -> PathFollower_Preview_1/10(CorneringStiffness_Tyres_Rear [N/rad])
  steering_ratio/1 -> PathFollower_Preview_1/11(steering_ratio[-])
  InitialVelocity/1 -> PathFollower_Preview_1/3(Initial Velocity [m/s])
  DesiredVelocity/1 -> PathFollower_Preview_1/4(Desired Velocity [m/s])
  Dynamics_Simple/1(State) -> [State], STATE_BMW_X5_SUV_1_rc/1
  [State] -> State2PathFollowerCnv/1(State BUS)
  State2PathFollowerCnv/1(Yaw rate [deg/s]) -> PathFollower_Preview_1/8(Yaw rate [deg/s])
  State2PathFollowerCnv/2(velocity [m/s]) -> PathFollower_Preview_1/5(velocity [m/s])  "veolcity"
  State2PathFollowerCnv/3(position x,y,Y [m,m,deg]) -> PathFollower_Preview_1/2(position x,y,Y [m,m,deg])
  PathFollower_Preview_1/1(delta_steerwheel [deg]) -> Subsystem/13(In13), Dynamics_Simple/1(DeltaSteer_[deg])  "steer[deg]"
  PathFollower_Preview_1/2(throttle [%]) -> Dynamics_Simple/2(Throttle)
  PathFollower_Preview_1/3(brake pressure [bar]) -> Dynamics_Simple/3(Brake)
  PathFollower_Preview_1/4(v0 [m/s]) -> Dynamics_Simple/4(Initial_Vx_[ms-1])
  PathFollower_Preview_1/5(Auto_GearShift) -> Dynamics_Simple/6(Auto_GearShift)
  Dynamics_Simple/3(Perf_Params) -> [Dynamics2PathFollower]
  FromDynamics2PathFollowerBusSelector/1 -> PathFollower_Preview_1/6(vx [m/s])  "<vx_[ms-1]>"
  FromDynamics2PathFollowerBusSelector/2 -> PathFollower_Preview_1/7(vy [m/s])  "<vy_[ms-1]>"
  [Dynamics2PathFollower] -> FromDynamics2PathFollowerBusSelector/1
  ? -> Dynamics_Simple/5(AutoManual_OnOff)
  ? -> Dynamics_Simple/7(Manual_GearShift)
  Dynamics_Simple/2(Vx [m s-1]) -> ?
  ? -> PathFollower_Preview_1/1(ActorOffset_Left(+) / Right(-) [m])
  PathFollower_Preview_1/6(Actor/Traj_distance [m]) -> Terminator_5/1
  PathFollower_Preview_1/7(Actor/Traj_angle [deg]) -> Terminator_6/1
  SELF_Demux/9(GPS alt [m]) -> Terminator_7/1  "GPS"
  Blank Message7/1 -> Bus Assignment7/1
  Divide1/1 -> Bus Assignment7/9
  Blank Message1/1 -> Bus Assignment1/1
  Data Type Conversion1/1 -> Bus Assignment1/3
  Constant15/1 -> Divide/2
  Divide/1 -> Bus Assignment7/8
  Bus Selector/13 -> Divide1/1  "<steer[deg]>"
  Constant16/1 -> Divide1/2
  Blank Message19/1 -> Bus Assignment19/1
  Subsystem10/2(Out2) -> Data Type Conversion92/1, Data Type Conversion91/1, Bus Assignment19/2, Data Type Conversion90/1, Bus Assignment1/30, Data Type Conversion1/1, Bus Assignment1/2, Subsystem7/1(In1), Bus Assignment7/17, Display2/1
  Data Type Conversion90/1 -> Bus Assignment19/3
  Constant348/1 -> Bus Assignment21/6
  Constant346/1 -> Bus Assignment21/4
  Constant347/1 -> Bus Assignment21/5
  Bus Assignment21/1 -> Bus Assignment19/4
  Subsystem4/1(Out1) -> Bus Assignment21/1
  Subsystem4/2(Out2) -> Bus Assignment21/2
  Subsystem4/3(Out3) -> Bus Assignment21/3
  Subsystem5/8(Out8) -> Bus Assignment7/35, Bus Assignment7/34, Bus Assignment7/29
  Subsystem5/1(Out1) -> Bus Assignment7/21
  Subsystem5/2(Out2) -> Bus Assignment7/22
  Subsystem5/3(Out3) -> Bus Assignment7/23
  Subsystem5/4(Out4) -> Bus Assignment7/24
  Subsystem5/5(Out5) -> Bus Assignment7/25
  Subsystem5/6(Out6) -> Bus Assignment7/26
  Subsystem5/7(Out7) -> Bus Assignment7/27
  Subsystem5/9(Out9) -> Bus Assignment7/28
  Subsystem5/10(Out10) -> Bus Assignment7/30
  Subsystem5/11(Out11) -> Bus Assignment7/31
  Subsystem6/1(Out1) -> Bus Assignment7/36
  Subsystem7/1(Out1) -> Bus Assignment7/10
  Subsystem7/2(Out2) -> Bus Assignment7/11
  Subsystem7/3(Out3) -> Bus Assignment7/12
  Subsystem7/4(Out4) -> Bus Assignment7/13
  Subsystem7/5(Out5) -> Bus Assignment7/14
  Subsystem7/6(Out6) -> Bus Assignment7/15
  Subsystem7/7(Out7) -> Bus Assignment7/16
  Subsystem7/8(Out8) -> Bus Assignment7/18
  Subsystem8/1(Out1) -> Bus Assignment7/2
  Subsystem9/1(Out1) -> Bus Assignment7/5
  Subsystem9/2(Out2) -> Bus Assignment7/6
  Data Type Conversion92/1 -> Bus Assignment22/3
  PolygonPoint/1 -> Bus Assignment23/9
  Blank Message23/1 -> Bus Assignment23/1
  Constant352/1 -> Data Type Conversion95/1
  Constant358/1 -> Data Type Conversion97/1
  "Position "/1 -> Bus Assignment23/3
  Blank Message24/1 -> PolygonPoint/1, Velocity/1, "Position "/1
  Data Type Conversion91/1 -> Bus Assignment22/2
  Velocity/1 -> Bus Assignment23/5
  Sum6/1 -> Bus Assignment23/8
  Constant361/1 -> Data Type Conversion93/1
  Blank Message22/1 -> Bus Assignment22/1
  Data Type Conversion93/1 -> Bus Assignment22/4, Bus Assignment22/5, Bus Assignment22/6
  Data Type Conversion94/1 -> Bus Assignment23/2
  Blank Message25/1 -> Bus Assignment/1
  Abs/1 -> Bus Assignment23/7
  [Car_value] -> Bus Selector6/1
  Bus Selector6/1 -> Sum/2  "<x>"
  Sum/1 -> PolygonPoint/2, "Position "/2
  Bus Selector6/2 -> Sum1/2  "<y>"
  Bus Selector6/3 -> Sum2/2  "<z>"
  Sum2/1 -> PolygonPoint/4, "Position "/4
  Sum1/1 -> PolygonPoint/3, "Position "/3
  [Dynamic] -> Bus Selector7/1
  Bus Selector5/14 -> Sum5/1  "<DopplerVelocityZ[ms-1]>"
  Bus Selector7/1 -> Sum3/2  "<vx_[ms-1]>"
  Bus Selector7/2 -> Sum4/2  "<vy_[ms-1]>"
  Bus Selector7/3 -> Sum5/2  "<vz_[ms-1]>"
  Sum3/1 -> Velocity/2
  Sum4/1 -> Velocity/3
  Sum5/1 -> Velocity/4
  Sum7/1 -> Abs/1
  Subsystem3/1(Out1) -> Bus Assignment23/6
  Subsystem3/2(Out2) -> Bus Assignment23/10
  Subsystem3/3(Out3) -> Bus Assignment23/11
  Subsystem3/4(Out4) -> Bus Assignment23/12
  Subsystem3/5(Out5) -> Bus Assignment23/13
  Subsystem3/6(Out6) -> Bus Assignment23/14
  Subsystem3/7(Out7) -> Bus Assignment23/15
  Bus Selector2/1 -> ?  "<Object ID>"
  Bus Assignment23/1 -> Bus Assignment/2
  Data Type Conversion97/1 -> Bus Assignment/3
  Bus Assignment22/1 -> Bus Assignment/4
  Data Type Conversion95/1 -> Bus Assignment/5
  PointCloudSensor_1/1 -> PointCloudSensor_1_WorldPos_Demux/1(In1)
  PointCloudSensor_1_WorldPos_Demux/1(X) -> PointCloudSensor_1_Display/1
  PointCloudSensor_1_WorldPos_Demux/2(Y) -> PointCloudSensor_1_Display/2
  PointCloudSensor_1_WorldPos_Demux/3(Z) -> PointCloudSensor_1_Display/3
  MATLAB Function1/2(Qx) -> Bus Assignment1/7
  MATLAB Function1/3(Qy) -> Bus Assignment1/8
  MATLAB Function1/4(Qz) -> Bus Assignment1/9
  MATLAB Function1/1(Qw) -> Bus Assignment1/10
  Bus Selector3/3 -> Discrete Derivative5/1, Bus Assignment1/19  "<AngularVelocityYaw>"
  Discrete Derivative/1 -> Bus Assignment1/21
  Discrete Derivative1/1 -> Bus Assignment1/22
  Discrete Derivative2/1 -> Bus Assignment1/23
  Discrete Derivative3/1 -> Bus Assignment1/24
  Discrete Derivative4/1 -> Bus Assignment1/25
  Discrete Derivative5/1 -> Bus Assignment1/26
  MATLAB Function2/1(Ex) -> Bus Assignment1/27
  MATLAB Function2/2(Ey) -> Bus Assignment1/28
  MATLAB Function2/3(Ez) -> Bus Assignment1/29
  Bus Assignment7/1 -> Publish5/1
  Subsystem10/1(Out1) -> Display1/1
  Bus Assignment1/1 -> Publish1/1
  Bus Assignment19/1 -> Publish2/1
  Bus Assignment/1 -> Publish3/1
  Bus Selector6/4 -> ?  "<Rotx>"
  Bus Selector6/6 -> ?  "<Rotz>"
  Bus Selector6/5 -> ?  "<Roty>"
  [State] -> Bus Selector3/1
  Bus Selector3/1 -> Discrete Derivative3/1, Bus Assignment1/17  "<AngularVelocityRoll>"
  Bus Selector3/2 -> Discrete Derivative4/1, Bus Assignment1/18  "<AngularVelocityPitch>"
  MATLAB Function/1(RotationMatrix) -> Coordinate Transformation Conversion/1, Coordinate Transformation Conversion1/1
  [Car_value] -> Bus Selector4/1
  Bus Selector4/2 -> MATLAB Function/2(Roty)  "<Roty>"
  Bus Selector4/1 -> MATLAB Function/1(Rotx)  "<Rotx>"
  Bus Selector4/3 -> MATLAB Function/3(Rotz)  "<Rotz>"
  Coordinate Transformation Conversion1/1 -> MATLAB Function2/1(Euler)
  Coordinate Transformation Conversion/1 -> MATLAB Function1/1(Quat)
  Constant1/1 -> Data Type Conversion2/1
  Data Type Conversion2/1 -> Bus Assignment19/5
  Constant2/1 -> Cast To Boolean/1
  Cast To Boolean/1 -> Bus Assignment19/6

== system Original_example1_cs/BoundingRectangle_1 ==
  Sensor : S-Function  FunctionName=sfun_BRS  Parameters=sensorID, detectableObjects, timestep  SFunctionDeploymentMode=off  EnableBusSupport=off  mask(PreScan Source Block: Bounding Rectangle Sensor){sensorID=66, detectableObjects=32, timestep=1/20}
      mask prompts: sensorID "Sensor ID"; detectableObjects "Max detectable objects:"; timestep "MATLAB timestep:"
      mask help: The Bounding Rectangle Sensor provides information of whereabouts of objects in images.
      mask Help: eval('openHelp(1462)')
      mask Display: image(imread('BoundingRectangleSensorSL.png'))
  BoundingRectangle_1 : Outport  Tag=outport/BRS  OutDataTypeStr=Bus: PRESCAN_BRS_MESSAGE  PortDimensions=32  SampleTime=1/20
  wires:
  Sensor/1 -> BoundingRectangle_1/1
